simulink subsystem "MCuC_CAN"  (R2023b)
settings: Solver=VariableStepAuto  StartTime=0.0  StopTime=10.0  RelTol=1e-3
libraries: msbUtilities x1
settings Model: Creator=nickj  LastModifiedBy=heyka

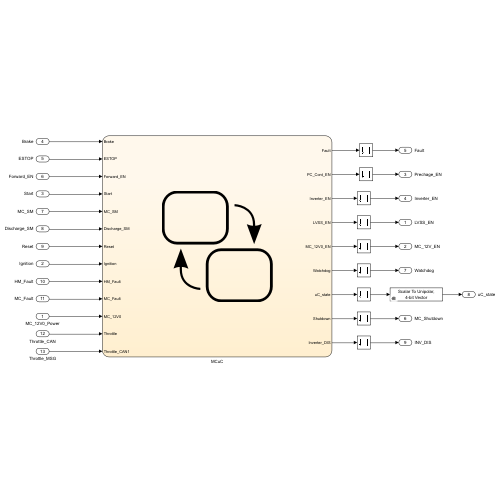
[thumbnail: Simulink's stored preview of the top-level diagram]
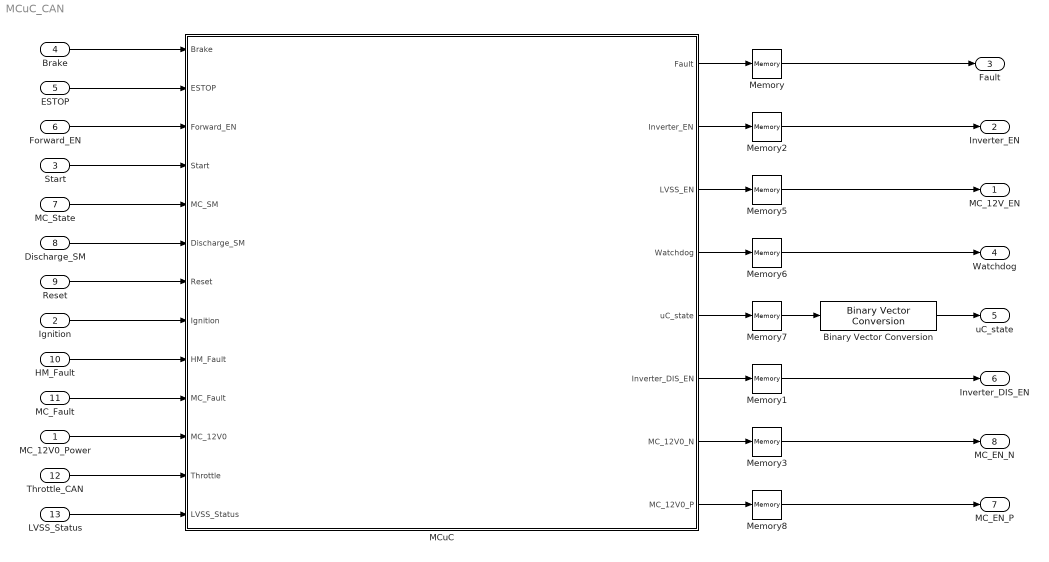
== system MCuC_CAN ==
  MC_12V0_Power : Inport
  Ignition : Inport  Port=2
  Start : Inport  Port=3
  Brake : Inport  Port=4
  ESTOP : Inport  Port=5
  Forward_EN : Inport  Port=6
  MC_State : Inport  Port=7
  Discharge_SM : Inport  Port=8
  Reset : Inport  Port=9
  HM_Fault : Inport  Port=10
  MC_Fault : Inport  Port=11
  Throttle_CAN : Inport  Port=12
  LVSS_Status : Inport  Port=13
  Binary Vector Conversion : msbUtilities/Binary Vector Conversion  LabelModeActiveChoice=To Unipolar  Convert=Scalar to binary-coded vector  Encoding=Unipolar (magnitude)  InputLength=8  InputReverse=LSB at index 1  OutputLength=4  OutputReverse=LSB at index 1  DataType=double
  MCuC : Stateflow chart  TreatAsAtomicUnit=on
      settings: PortSchema="{\"entries\":[{\"content\":{\"sides\":[{\"content\":{\"connectorIds\":[\"In1\",\"In2\",\"In3\",\"In5\",\"In6\",\"In7\",\"In8\",\"In4\",\"In9\",\"In10\",\"In11\",\"In12\",\"In13\"]},\"type\":\"ConnectorPlacement.EquallySpacedRectSide\",\"uuid\":\"d1510c73-f1c7-4e03-bb6c-bda7856f993e\"},{\"content\":{\"connectorIds\":[\"Out1\",\"Out2\",\"Out3\",\"Out4\",\"Out5\",\"Out6\",\"Out7\",\"Out8\"],\"side\":\"RIGHT\"},\"type\":\"ConnectorPlacement.EquallySpacedRectSide\",\"uuid\":\"1a7878c4-a817-4ca0-b21c-0429e82bb9d7\"},{\"content\":{\"side\":\"TOP\"},\"type\":\"ConnectorPlacement.EquallySpacedRectSide\",\"uuid\":\"ed9f2701-7044-4bb4-9c0b-b9cf9840e69e\"}]},\"type\":\"ConnectorPlacement.EquallySpacedConnector\",\"uuid\":\"4ceb8e7d-629c-4438-88a9-aa3016537644\"}],\"packageUris\":[\"http://schema.mathworks.com/mf0/Connector/R2020b\"],\"version\":\"1.0\"}"
  Memory{,1..3,5..8} (8 alike) : Memory
  MC_12V_EN : Outport
  Inverter_EN : Outport  Port=2
  Fault : Outport  Port=3
  Watchdog : Outport  Port=4
  uC_state : Outport  Port=5
  Inverter_DIS_EN : Outport  Port=6
  MC_EN_P : Outport  Port=7
  MC_EN_N : Outport  Port=8
  wires:
  Brake/1 -> MCuC/1(Brake)
  Discharge_SM/1 -> MCuC/7(Discharge_SM)
  ESTOP/1 -> MCuC/2(ESTOP)
  Forward_EN/1 -> MCuC/3(Forward_EN)
  Start/1 -> MCuC/5(Start)
  Reset/1 -> MCuC/8(Reset)
  MC_State/1 -> MCuC/6(MC_SM)
  Ignition/1 -> MCuC/4(Ignition)
  HM_Fault/1 -> MCuC/9(HM_Fault)
  Memory6/1 -> Watchdog/1
  MC_Fault/1 -> MCuC/10(MC_Fault)
  MCuC/1(Fault) -> Memory/1
  MCuC/2(Inverter_EN) -> Memory2/1
  Memory2/1 -> Inverter_EN/1
  MCuC/3(LVSS_EN) -> Memory5/1
  MCuC/4(Watchdog) -> Memory6/1
  MCuC/5(uC_state) -> Memory7/1
  Memory/1 -> Fault/1
  Memory5/1 -> MC_12V_EN/1
  MC_12V0_Power/1 -> MCuC/11(MC_12V0)
  Throttle_CAN/1 -> MCuC/12(Throttle)
  Memory7/1 -> Binary Vector Conversion/1
  Binary Vector Conversion/1 -> uC_state/1
  MCuC/6(Inverter_DIS_EN) -> Memory1/1
  MCuC/7(MC_12V0_N) -> Memory3/1
  MCuC/8(MC_12V0_P) -> Memory8/1
  Memory1/1 -> Inverter_DIS_EN/1
  Memory3/1 -> MC_EN_N/1
  Memory8/1 -> MC_EN_P/1
  LVSS_Status/1 -> MCuC/13(LVSS_Status)

== stateflow chart MCuC_CAN/MCuC ==
  state MCuC
    state MCuC_Logic [parallel]
      settings: executionOrder=1
      state ESTOP
        entry:
        uC_state = 7;
        LVSS_EN = 0;
        ESTOP_activated = 0;
      state MC_Off
        entry:
        LVSS_EN = 0;
        uC_state = 0;
        uncharged = 1;
        Inverter_EN = 0;
        Inverter_DIS_EN = 0;
      state MC_Discharging
        entry:
        uC_state = 5;
        MC_12V0_P = 0;
        MC_12V0_N = 1;
        exit:
        MC_12V0_P = 0;
        MC_12V0_N = 0;
      state Fault
        entry:
        uC_state = 6;
        Fault = 1;
        exit:
        Fault = 0;
      state Contactor_Open
        entry:
        Inverter_EN = 0;
        Inverter_DIS_EN = 1;
        uC_state = 4;
      state MC_Init
        entry:
        uncharged = 0;
        Inverter_EN = 0;
        uC_state = 1;
        LVSS_EN = 1;
        MC_12V0_P = 1;
        MC_12V0_N = 0;
        exit:
        MC_12V0_P = 0;
        MC_12V0_N = 0;
      state MC_Active
        entry:
        Inverter_EN = 1;
        uC_state = 3;
      state Reset
        entry:
        uC_state = 8;
      state Contactor_Closed
        entry:
        uC_state = 2;
        Inverter_EN = 0;
      (default) -> MC_Off
      ESTOP -> MC_Off : [ESTOP == 0]
      MCuC_Logic -> ESTOP [order 3] : [ESTOP == 1 && uncharged == 1 && Reset == 0]
      Fault -> MC_Off : [MC_12V0 == 0 && Ignition == 0]
      MC_Discharging -> MC_Off : [Discharge_SM == 4 && LVSS_Status == 0]
      Reset -> MC_Off : [MC_12V0 == 0 && Ignition == 0]
      MC_Off -> MC_Init : [Ignition == 1]
      Contactor_Open -> MC_Discharging : [Discharge_SM == 3]
      MCuC_Logic -> Fault [order 4] : [HM_Fault == 1 && Ignition == 1]
      MCuC_Logic -> Fault [order 2] : [MC_Fault == 1 && Ignition == 1]
      MCuC_Logic -> Contactor_Open [order 1] : [ESTOP == 1 && uncharged == 0 && ESTOP_activated == 0]{ESTOP_activated = 1}
      MC_Init -> Contactor_Open [order 1] : [Ignition == 0]
      MC_Init -> Contactor_Closed [order 2] : [MC_SM == 4 && LVSS_Status == 1]
      Contactor_Closed -> Contactor_Open [order 2] : [Ignition == 0]
      MC_Active -> Contactor_Open [order 2] : [Ignition == 0]
      Contactor_Closed -> MC_Active [order 1] : [Start == 1 && Forward_EN == 1 && Brake == 1 && Throttle == 0]
      MCuC_Logic -> Reset [order 5] : [Reset == 1 && Ignition == 1]
      MC_Active -> Contactor_Closed [order 1] : [Forward_EN == 0]
    state Watchdog [parallel]
      settings: executionOrder=2
      state WD0
        entry:
        Watchdog = 0;
      state WD1
        entry:
        Watchdog = 1;
      (default) -> WD0
      WD0 -> WD1 : after(.5, sec)
      WD1 -> WD0
  data: Fault output =0; Brake input; ESTOP input; Forward_EN input; Ignition input; Start input; MC_SM input; Inverter_EN output =0; LVSS_EN output =0; Discharge_SM input; Reset input; Watchdog output =0; uC_state output; uncharged local; ESTOP_activated local =0; HM_Fault input; MC_Fault input; MC_12V0 input; Throttle input; LVSS_Status input; Inverter_DIS_EN output =0; MC_12V0_N output =0; MC_12V0_P output =0
